simulink model "HLAblock"  (R2019b)
settings: Solver=FixedStepDiscrete  StartTime=0.0  StopTime=600000  FixedStep=1  RelTol=1e-3
settings Model: Creator=k-110-04  LastModifiedBy=k-110-04
settings SolverCC: AlgebraicLoopSolver=LineSearch
settings OptimizationCC: DefaultParameterBehavior=Inlined  EnhancedBackFolding=on  PassReuseOutputArgsThreshold=0  OptimizeBlockOrder=speed  DifferentSizesBufferReuse=on  OptimizationCustomize=off
settings DebuggingCC: ParameterTunabilityLossMsg=error  ModelReferenceDataLoggingMessage=none  SFUnexpectedBacktrackingDiag=warning  SFNoUnconditionalDefaultTransitionDiag=warning
settings HardwareCC: ProdBitPerLong=64  ProdHWDeviceType=Intel->x86-64 (Linux 64)  TargetBitPerLong=64  TargetBitPerPointer=64  TargetBitPerSizeT=64  TargetBitPerPtrDiffT=64  TargetLargestAtomicFloat=Float  TargetIntDivRoundTo=Zero  TargetEndianess=LittleEndian  TargetWordSize=64  TargetHWDeviceType=Intel->x86-64 (Linux 64)
settings SFSimCC: MATLABDynamicMemAlloc=off
settings RTWCC: Description=Generic Real-Time Target  GenerateReport=on  RTWVerbose=off  RTWUseSimCustomCode=on  Toolchain=GNU gcc/g++ | gmake (64-bit Linux)  BuildConfiguration=Specify  LaunchReport=on  TargetLang=C++  CheckMdlBeforeBuild=Warning
settings CodeAppCC: ForceParamTrailComments=on  OperatorAnnotations=on  EnableCustomComments=on
settings GRTTargetCC: TargetLangStandard=C++03 (ISO)  MatFileLogging=off  MultiInstanceERTCode=on  CodeInterfacePackaging=C++ class

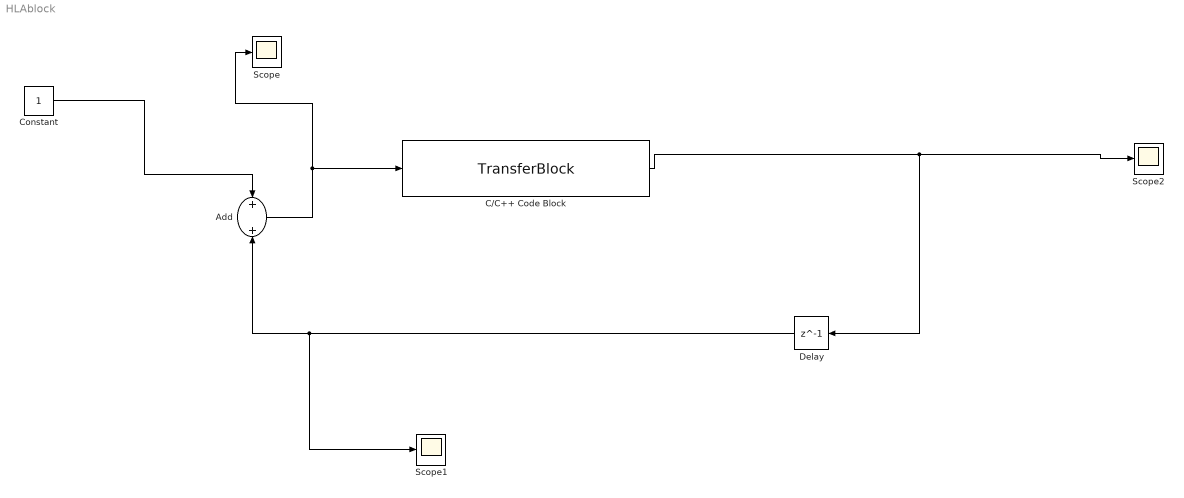
== system HLAblock ==
  Add : Sum
  C/C++ Code Block : S-Function  InitFcn=try, set_param(gcb,'FunctionName','TransferBlock'), end  FunctionName=TransferBlock  Parameters=1  SFunctionModules=TransferBlock_wrapper BaseFederate Logger SimFederate BasicException Tools  SFunctionDeploymentMode=off  EnableBusSupport=off  mask(S-Function Builder){}
      mask help: Simulink:masks:SFunctionBuilder_MD
      mask init:
      | val = [[.9  0.75 0.75 1 1 .9 .9 1]',[1 1 0.75 0.75 .9 .9 1 .9]'];try , sys = get_param(gcb,'SfunBuilderFcnName');if isempty(sys), sys = get_param(gcb,'FunctionName'); end,catch, sys = get_param(gcb,'FunctionName'); end
      settings: CopyFcn=set_param(gcbh,'LinkStatus','none')  PreSaveFcn=try, set_param(gcb,'FunctionName','TransferBlock'), end  OpenFcn=sfunctionwizard(gcbh)
      mask Display: plot(val(:,1),val(:,2)),disp(sys), port_label('input',1,'X'), port_label('output',1,'Y')
  Constant : Constant
  Delay : Delay  DelayLength=1
  Scope : Scope
  Scope1 : Scope
  Scope2 : Scope
  wires:
  C/C++ Code Block/1 -> Delay/1, Scope2/1
  Delay/1 -> Scope1/1, Add/2
  Constant/1 -> Add/1
  Add/1 -> Scope/1, C/C++ Code Block/1
